simulink model "MotorSim"  (R2016b)
settings: Solver=VariableStepAuto  StartTime=0.0  StopTime=10  RelTol=1e-3
values from neighbouring files (symbols this model uses):
  d_min = 1    [MotorParam.m]
  e_max = 18    [MotorParam.m]
  g = 9.8    [MotorParam.m]    (also in PumpParam.m)
  incline = 0    [MotorParam.m]
  J = 0.02    [MotorParam.m]    (also in PumpParam.m)
  Kf = 0.2    [MotorParam.m]    (also in PumpParam.m)
  Ki = 1    [MotorParam.m]
  Km = 1    [MotorParam.m]    (also in PumpParam.m)
  Kp = 1    [MotorParam.m]
  L = 0.5    [MotorParam.m]    (also in PumpParam.m)
  M = 5    [MotorParam.m]
  mu = 0.8    [MotorParam.m]
  R = 2.0    (= 2)    [MotorParam.m]    (also in PumpParam.m)
  r_w = 0.05    [MotorParam.m]
  t_loss = 0    [MotorParam.m]
  w_ref = w_rpm*(pi/30)    (= 31.4159265359)    [MotorParam.m]
undefined symbols (not defined in the file or in its folder): Tstall, w_noload
libraries: simulink x3
settings Model: Creator=curtm  LastModifiedBy=curtm

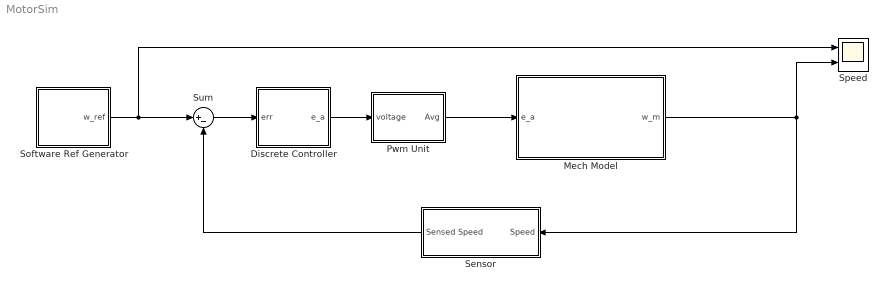
== system MotorSim ==
  Discrete Controller : Subsystem
  Mech Model : Subsystem
  Pwm Unit : Subsystem
  Sensor : Subsystem
  Software Ref Generator : Subsystem
  Speed : Scope  NumInputPorts=2
  Sum : Sum  Inputs=|+-
  wires:
  Mech Model/1(w_m) -> Speed/2, Sensor/1(Speed)
  Discrete Controller/1(e_a) -> Pwm Unit/1(voltage)
  Software Ref Generator/1(w_ref) -> Speed/1, Sum/1
  Sum/1 -> Discrete Controller/1(err)
  Pwm Unit/1(Avg) -> Mech Model/1(e_a)
  Sensor/1(Sensed Speed) -> Sum/2

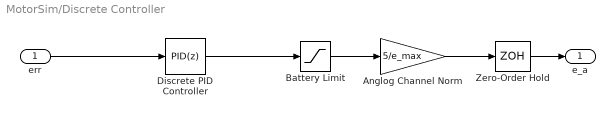
== system MotorSim/Discrete Controller ==
  err : Inport
  Anglog Channel Norm : Gain  Gain=5/e_max
  Battery Limit : Saturate  UpperLimit=e_max  LowerLimit=-e_max
  Discrete PID Controller : simulink/Continuous/PID Controller  Controller=PID  TimeDomain=Discrete-time  SampleTime=-1  IntegratorMethod=Forward Euler  FilterMethod=Forward Euler  Form=Parallel  UseFilter=on  ControllerParametersSource=internal  P=Kp  I=Ki  D=0  N=100  InitialConditionSource=internal  InitialConditionForIntegrator=0  InitialConditionForFilter=0  ExternalReset=none  LimitOutput=off  UpperSaturationLimit=inf  LowerSaturationLimit=-inf  LinearizeAsGain=off  AntiWindupMode=none  Kb=1  TrackingMode=off  Kt=1  PParamMin=[]  PParamMax=[]  IParamMin=[]  IParamMax=[]  DParamMin=[]  DParamMax=[]  NParamMin=[]  NParamMax=[]  KbParamMin=[]  KbParamMax=[]  KtParamMin=[]  KtParamMax=[]  POutMin=[]  POutMax=[]  IOutMin=[]  IOutMax=[]  DOutMin=[]  DOutMax=[]  NOutMin=[]  NOutMax=[]  KbOutMin=[]  KbOutMax=[]  KtOutMin=[]  KtOutMax=[]  IntegratorOutMin=[]  IntegratorOutMax=[]  FilterOutMin=[]  FilterOutMax=[]  SumOutMin=[]  SumOutMax=[]  SumI1OutMin=[]  SumI1OutMax=[]  SumI2OutMin=[]  SumI2OutMax=[]  SumI3OutMin=[]  SumI3OutMax=[]  SumDOutMin=[]  SumDOutMax=[]  SaturationOutMin=[]  SaturationOutMax=[]  IntegratorContinuousStateAttributes=''  IntegratorStateMustResolveToSignalObject=off  IntegratorRTWStateStorageClass=Auto  FilterContinuousStateAttributes=''  FilterStateMustResolveToSignalObject=off  FilterRTWStateStorageClass=Auto  DifferentiatorICPrevScaledInput=0  DifferentiatorOutMin=[]  DifferentiatorOutMax=[]
  Zero-Order Hold : ZeroOrderHold  SampleTime=-1
  e_a : Outport
  wires:
  Discrete PID Controller/1 -> Battery Limit/1
  err/1 -> Discrete PID Controller/1
  Battery Limit/1 -> Anglog Channel Norm/1
  Anglog Channel Norm/1 -> Zero-Order Hold/1
  Zero-Order Hold/1 -> e_a/1

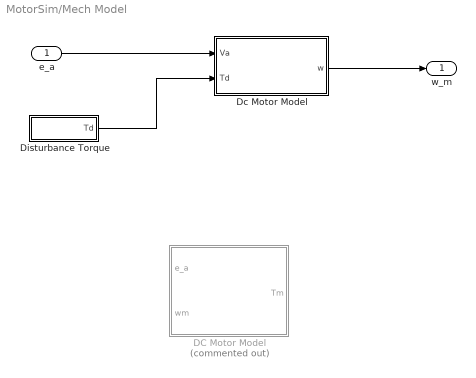
== system MotorSim/Mech Model ==
  e_a : Inport
  DC Motor Model : Subsystem  Commented=on
  Dc Motor Model : Subsystem
  Disturbance Torque : Subsystem
  w_m : Outport
  wires:
  e_a/1 -> Dc Motor Model/1(Va)
  Disturbance Torque/1(Td) -> Dc Motor Model/2(Td)
  Dc Motor Model/1(w) -> w_m/1

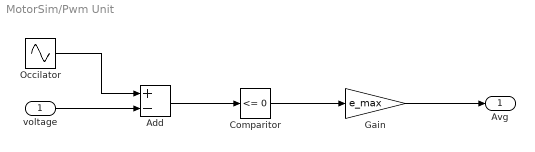
== system MotorSim/Pwm Unit ==
  voltage : Inport
  Add : Sum  Inputs=+-
  Comparitor : simulink/Logic and Bit Operations/Compare To Zero  relop=<=  OutDataTypeStr=boolean
  Gain : Gain  Gain=e_max
  Occilator : Sin  Amplitude=5  SampleTime=0
  Avg : Outport
  wires:
  Occilator/1 -> Add/1
  voltage/1 -> Add/2
  Add/1 -> Comparitor/1
  Comparitor/1 -> Gain/1
  Gain/1 -> Avg/1

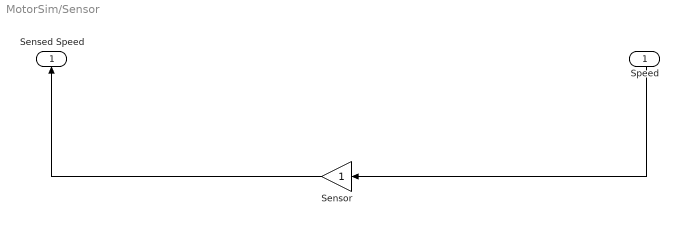
== system MotorSim/Sensor ==
  Speed : Inport
  Sensor : Gain
  Sensed Speed : Outport
  wires:
  Speed/1 -> Sensor/1
  Sensor/1 -> Sensed Speed/1

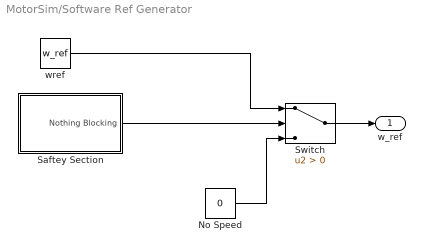
== system MotorSim/Software Ref Generator ==
  No Speed : Constant  Value=0
  Saftey Section : Subsystem
  Switch : Switch  Criteria=u2 > Threshold
  wref : Constant  Value=w_ref
  w_ref : Outport
  wires:
  Switch/1 -> w_ref/1
  wref/1 -> Switch/1
  No Speed/1 -> Switch/3
  Saftey Section/1(Nothing Blocking) -> Switch/2

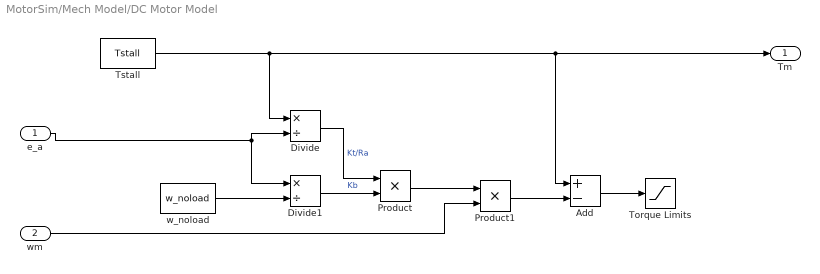
== system MotorSim/Mech Model/DC Motor Model ==
  e_a : Inport
  wm : Inport  Port=2
  Add : Sum  Inputs=+-
  Divide : Product  Inputs=*/
  Divide1 : Product  Inputs=*/
  Product : Product
  Product1 : Product
  Torque Limits : Saturate  UpperLimit=Tstall  LowerLimit=-Tstall
  Tstall : Constant  Value=Tstall
  w_noload : Constant  Value=w_noload
  Tm : Outport
  wires:
  Divide1/1 -> Product/2  "Kb"
  Divide/1 -> Product/1  "Kt/Ra"
  Tstall/1 -> Tm/1, Add/1, Divide/1
  Product1/1 -> Add/2
  e_a/1 -> Divide/2, Divide1/1
  w_noload/1 -> Divide1/2
  wm/1 -> Product1/2
  Product/1 -> Product1/1
  Add/1 -> Torque Limits/1

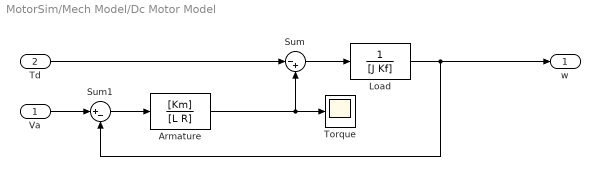
== system MotorSim/Mech Model/Dc Motor Model ==
  Va : Inport
  Td : Inport  Port=2
  Armature : TransferFcn  Numerator=[Km]  Denominator=[L R]
  Load : TransferFcn  Denominator=[J Kf]
  Sum : Sum  Inputs=|-+
  Sum1 : Sum  Inputs=|+-
  Torque : Scope
  w : Outport
  wires:
  Va/1 -> Sum1/1
  Sum1/1 -> Armature/1
  Armature/1 -> Torque/1, Sum/2
  Td/1 -> Sum/1
  Load/1 -> w/1, Sum1/2
  Sum/1 -> Load/1

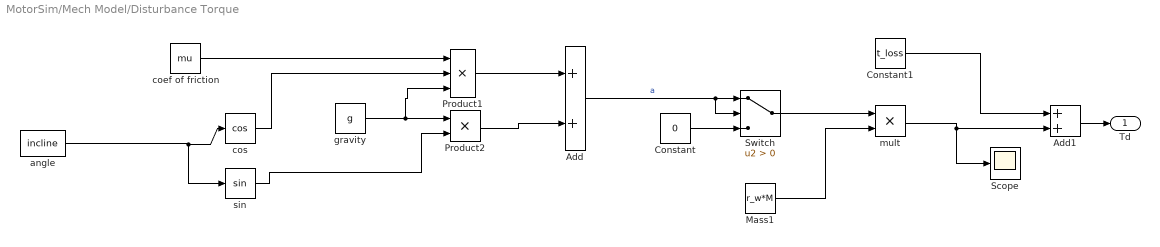
== system MotorSim/Mech Model/Disturbance Torque ==
  Add : Sum
  Add1 : Sum
  Constant : Constant  Value=0
  Constant1 : Constant  Value=t_loss
  Mass1 : Constant  Value=r_w*M
  Product1 : Product  Inputs=3
  Product2 : Product
  Scope : Scope
  Switch : Switch  Criteria=u2 > Threshold
  angle : Constant  Value=incline
  coef of friction : Constant  Value=mu
  cos : Trigonometry  Operator=cos
  gravity : Constant  Value=g
  "mult " : Product  Inputs=**
  sin : Trigonometry
  Td : Outport
  wires:
  coef of friction/1 -> Product1/1
  gravity/1 -> Product1/3, Product2/1
  Product1/1 -> Add/1
  Product2/1 -> Add/2
  cos/1 -> Product1/2
  Add/1 -> Switch/2, Switch/1  "a"
  angle/1 -> cos/1, sin/1
  sin/1 -> Product2/2
  Constant/1 -> Switch/3
  Switch/1 -> "mult "/1
  Mass1/1 -> "mult "/2
  "mult "/1 -> Add1/2, Scope/1
  Add1/1 -> Td/1
  Constant1/1 -> Add1/1

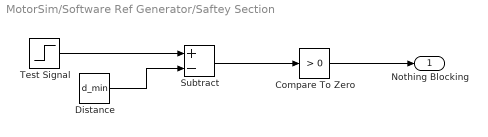
== system MotorSim/Software Ref Generator/Saftey Section ==
  Compare To Zero : simulink/Logic and Bit Operations/Compare To Zero  relop=>  OutDataTypeStr=boolean
  Distance : Constant  Value=d_min
  Subtract : Sum  Inputs=+-
  "Test Signal " : Step  Time=0  After=12  SampleTime=0
  Nothing Blocking : Outport
  wires:
  Compare To Zero/1 -> Nothing Blocking/1
  "Test Signal "/1 -> Subtract/1
  Subtract/1 -> Compare To Zero/1
  Distance/1 -> Subtract/2
